simulink model "ExternalController"  (R2019b)
settings: Solver=FixedStepAuto  StartTime=0.0  StopTime=1500  FixedStep=0.01  RelTol=1e-3
undefined symbols (not defined in the file): OP
settings Model: Creator=tarek  LastModifiedBy=tarek
settings ConfigComp: CovBoundaryAbsTol=1.0e-5

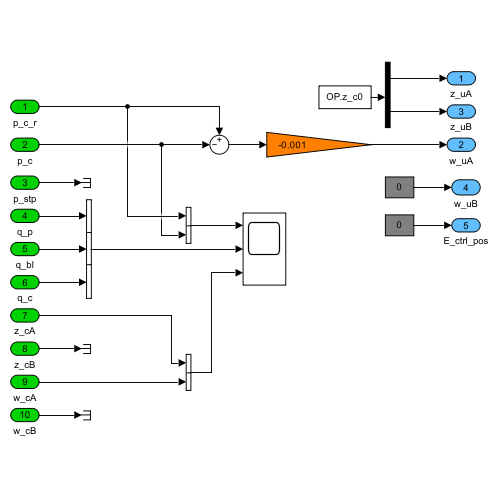
[thumbnail: Simulink's stored preview of the top-level diagram]
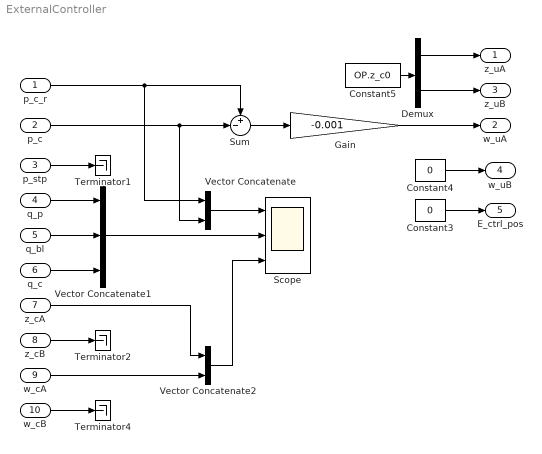
== system ExternalController ==
  p_c_r : Inport
  p_c : Inport  Port=2
  p_stp : Inport  Port=3
  q_p : Inport  Port=4
  q_bl : Inport  Port=5
  q_c : Inport  Port=6
  z_cA : Inport  Port=7
  z_cB : Inport  Port=8
  w_cA : Inport  Port=9
  w_cB : Inport  Port=10
  Constant3 : Constant  Value=0
  Constant4 : Constant  Value=0
  Constant5 : Constant  Value=OP.z_c0
  Demux : Demux  Outputs=2
  Gain : Gain  Gain=-0.001
  Scope : Scope  NumInputPorts=3
  Sum : Sum  Inputs=+-|
  Terminator1 : Terminator
  Terminator2 : Terminator
  Terminator4 : Terminator
  Vector Concatenate : Concatenate
  Vector Concatenate1 : Concatenate  NumInputs=3
  Vector Concatenate2 : Concatenate
  z_uA : Outport
  w_uA : Outport  Port=2
  z_uB : Outport  Port=3
  w_uB : Outport  Port=4
  E_ctrl_pos : Outport  Port=5
  wires:
  Constant4/1 -> w_uB/1
  p_stp/1 -> Terminator1/1
  z_cA/1 -> Vector Concatenate2/1
  p_c_r/1 -> Vector Concatenate/1, Sum/1
  Gain/1 -> w_uA/1
  p_c/1 -> Vector Concatenate/2, Sum/2
  q_p/1 -> Vector Concatenate1/1
  Vector Concatenate1/1 -> Scope/2
  Vector Concatenate/1 -> Scope/1
  Sum/1 -> Gain/1
  Demux/2 -> z_uB/1
  q_bl/1 -> Vector Concatenate1/2
  z_cB/1 -> Terminator2/1
  w_cB/1 -> Terminator4/1
  Vector Concatenate2/1 -> Scope/3
  w_cA/1 -> Vector Concatenate2/2
  Demux/1 -> z_uA/1
  Constant3/1 -> E_ctrl_pos/1
  Constant5/1 -> Demux/1
  q_c/1 -> Vector Concatenate1/3
